simulink model "TorqueDistribution"  (R2024b)
settings: Solver=FixedStepDiscrete  StartTime=0.0  StopTime=1  FixedStep=0.001  RelTol=1e-3  EnableMultiTasking=on
undefined symbols (not defined in the file): MMotorMinAllowed, MTotalMinAllowed, rGearboxRatio, rTyreRadius
libraries: simulink x8
settings Model: DataDictionary=Master_Dictionary.sldd  EnableAccessToBaseWorkspace=off  Creator=torni  LastModifiedBy=oxbro
settings SolverCC: AlgebraicLoopSolver=TrustRegion
settings DataIOCC: ReturnWorkspaceOutputs=off
settings OptimizationCC: DefaultParameterBehavior=Inlined  EnhancedBackFolding=on  PassReuseOutputArgsAs=Individual arguments  ZeroExternalMemoryAtStartup=off  ZeroInternalMemoryAtStartup=off  MaxStackSize=512  OptimizeBlockOrder=speed  DifferentSizesBufferReuse=on  OptimizationCustomize=off  EfficientTunableParamExpr=on
settings DebuggingCC: ParameterTunabilityLossMsg=error  UnconnectedInputMsg=warning  UnconnectedOutputMsg=warning  UnconnectedLineMsg=warning  ArithmeticOperatorsInVariantConditions=warning
settings HardwareCC: ProdBitPerPointer=32  ProdBitPerSizeT=32  ProdBitPerPtrDiffT=32  ProdLargestAtomicInteger=Long  ProdLargestAtomicFloat=Double  ProdWordSize=32  ProdLongLongMode=on  ProdHWDeviceType=ARM Compatible->ARM Cortex-M
settings ModelReferenceCC: EnableRefExpFcnMdlSchedulingChecks=on
settings SFSimCC: MATLABDynamicMemAlloc=off  CustomCodeUndefinedFunction=UseInterfaceOnly
settings RTWCC: Description=Embedded Coder  SystemTargetFile=ert.tlc  HardwareBoard=STM32H7xx Based (Single-core)  TemplateMakefile=ert_default_tmf  CustomHeaderCode="#include \"stm32h7xx_ll_tim.h\""  CustomInitializer=LL_TIM_EnableCounter(TIM2);  Toolchain=GNU Tools for ARM Embedded Processors  GPUComputeCapability=3.5
settings CodeAppCC: ForceParamTrailComments=on  IgnoreCustomStorageClasses=off  OperatorAnnotations=on  SimulinkDataObjDesc=on  SFDataObjDesc=on  InsertBlockDesc=on
settings ERTTargetCC: TargetLangStandard=C99 (ISO)  CodeReplacementLibrary=ARM Cortex-M  ExtModeTransport=3  ExtModeStaticAlloc=on  ExtModeStaticAllocSize=2048  ExtModeMexFile=ext_xcp  ExtModeIntrfLevel=Level2 - Open

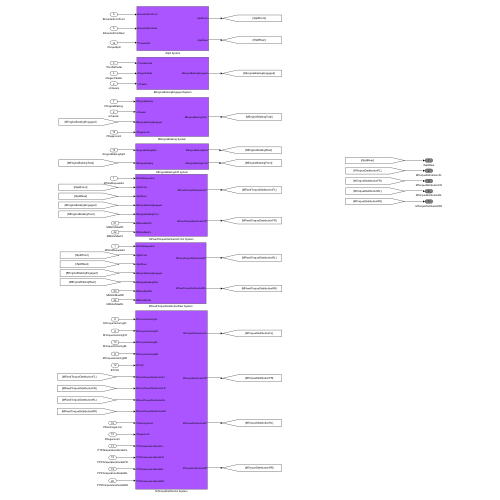
[thumbnail: Simulink's stored preview of the top-level diagram]
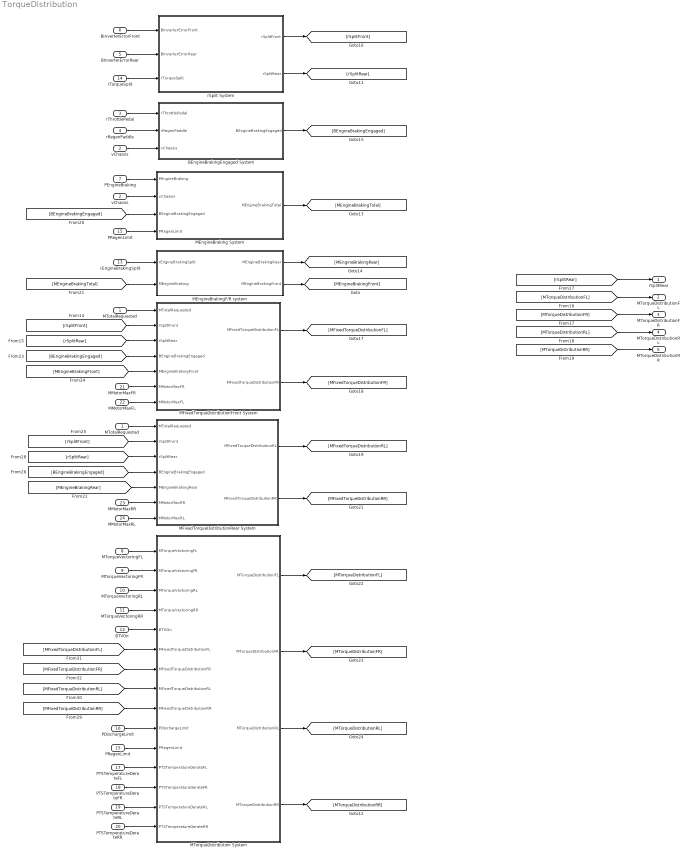
== system TorqueDistribution ==
  MTotalRequested : Inport  OutDataTypeStr=double
  vChassis : Inport  Port=2  OutDataTypeStr=double
  "rThrottlePedal " : Inport  Port=3  OutDataTypeStr=double
  rRegenPaddle : Inport  Port=4  OutDataTypeStr=double
  BInverterErrorRear : Inport  Port=5  OutDataTypeStr=boolean
  BInverterErrorFront : Inport  Port=6  OutDataTypeStr=boolean
  PEngineBraking : Inport  Port=7  OutDataTypeStr=double
  MTorqueVectoringFL : Inport  Port=8  OutDataTypeStr=double
  MTorqueVectoringFR : Inport  Port=9  OutDataTypeStr=double
  MTorqueVectoringRL : Inport  Port=10  OutDataTypeStr=double
  MTorqueVectoringRR : Inport  Port=11  OutDataTypeStr=double
  BTVOn : Inport  Port=12  OutDataTypeStr=boolean
  "rEngineBrakingSplit " : Inport  Port=13
  rTorqueSplit : Inport  Port=14  OutDataTypeStr=double
  PRegenLimit : Inport  Port=15  OutDataTypeStr=double
  PDischargeLimit : Inport  Port=16  OutDataTypeStr=double
  PTSTemperatureDerateFL : Inport  Port=17  OutDataTypeStr=double
  PTSTemperatureDerateFR : Inport  Port=18  OutDataTypeStr=double
  PTSTemperatureDerateRL : Inport  Port=19  OutDataTypeStr=double
  PTSTemperatureDerateRR : Inport  Port=20  OutDataTypeStr=double
  MMotorMaxFR : Inport  Port=21  OutDataTypeStr=double
  MMotorMaxFL : Inport  Port=22  OutDataTypeStr=double
  MMotorMaxRR : Inport  Port=23  OutDataTypeStr=double
  MMotorMaxRL : Inport  Port=24  OutDataTypeStr=double
  BEngineBrakingEngaged System : Subsystem
  MEngineBraking System : Subsystem
  MEngineBrakingF/R system : Subsystem
  MFixedTorqueDistributionFront System : Subsystem
  MFixedTorqueDistributionRear System : Subsystem
  MTorqueDistribution System : Subsystem
  "MTotalRequested " : InportShadow  OutDataTypeStr=double
  "PRegenLimit " : InportShadow  Port=15  OutDataTypeStr=double
  rSplit System : Subsystem
  "vChassis " : InportShadow  Port=2  OutDataTypeStr=double
  rSplitRear : Outport  OutDataTypeStr=double  VectorParamsAs1DForOutWhenUnconnected=off
  MTorqueDistributionFL : Outport  Port=2  OutDataTypeStr=double  VectorParamsAs1DForOutWhenUnconnected=off
  MTorqueDistributionFR : Outport  Port=3  OutDataTypeStr=double  VectorParamsAs1DForOutWhenUnconnected=off
  MTorqueDistributionRL : Outport  Port=4  OutDataTypeStr=double  VectorParamsAs1DForOutWhenUnconnected=off
  MTorqueDistributionRR : Outport  Port=5  OutDataTypeStr=double  VectorParamsAs1DForOutWhenUnconnected=off
  wires:
  [BEngineBrakingEngaged] -> MEngineBraking System/3(BEngineBrakingEngaged)
  vChassis/1 -> BEngineBrakingEngaged System/3(vChassis)
  MEngineBraking System/1("MEngineBrakingTotal ") -> [MEngineBrakingTotal]
  [MEngineBrakingRear] -> MFixedTorqueDistributionRear System/5("MEngineBrakingRear ")
  PEngineBraking/1 -> MEngineBraking System/1(PEngineBraking)
  [MEngineBrakingTotal] -> MEngineBrakingF/R system/2(MEngineBraking)
  MTorqueDistribution System/4(MTorqueDistributionRR) -> [MTorqueDistributionRR]
  [MFixedTorqueDistributionFR] -> MTorqueDistribution System/7(MFixedTorqueDistributionFR)
  MTorqueVectoringFR/1 -> MTorqueDistribution System/2(MTorqueVectoringFR)
  MFixedTorqueDistributionRear System/1(MFixedTorqueDistributionRL) -> [MFixedTorqueDistributionRL]
  [MTorqueDistributionRR] -> MTorqueDistributionRR/1
  "rEngineBrakingSplit "/1 -> MEngineBrakingF/R system/1(rEngineBrakingSplit)
  rTorqueSplit/1 -> rSplit System/3(rTorqueSplit)
  PRegenLimit/1 -> MEngineBraking System/4(PRegenLimit)
  [MTorqueDistributionFL] -> MTorqueDistributionFL/1
  [rSplitRear] -> MFixedTorqueDistributionRear System/3(rSplitRear)
  MEngineBrakingF/R system/1(MEngineBrakingRear) -> [MEngineBrakingRear]
  [rSplitRear] -> MFixedTorqueDistributionFront System/3(rSplitRear)
  BInverterErrorRear/1 -> rSplit System/2(BInverterErrorRear)
  [MTorqueDistributionRL] -> MTorqueDistributionRL/1
  MFixedTorqueDistributionFront System/2(MFixedTorqueDistributionFR) -> [MFixedTorqueDistributionFR]
  MTorqueDistribution System/3(MTorqueDistributionRL) -> [MTorqueDistributionRL]
  [BEngineBrakingEngaged] -> MFixedTorqueDistributionFront System/4(BEngineBrakingEngaged)
  [MFixedTorqueDistributionRR] -> MTorqueDistribution System/9(MFixedTorqueDistributionRR)
  [MTorqueDistributionFR] -> MTorqueDistributionFR/1
  MTorqueDistribution System/2(MTorqueDistributionFR) -> [MTorqueDistributionFR]
  MFixedTorqueDistributionRear System/2(MFixedTorqueDistributionRR) -> [MFixedTorqueDistributionRR]
  [rSplitFront] -> MFixedTorqueDistributionRear System/2(rSplitFront)
  BEngineBrakingEngaged System/1(BEngineBrakingEngaged) -> [BEngineBrakingEngaged]
  "MTotalRequested "/1 -> MFixedTorqueDistributionRear System/1(MTotalRequested)
  rRegenPaddle/1 -> BEngineBrakingEngaged System/2(rRegenPaddle)
  [rSplitFront] -> MFixedTorqueDistributionFront System/2(rSplitFront)
  MTotalRequested/1 -> MFixedTorqueDistributionFront System/1(MTotalRequested)
  "rThrottlePedal "/1 -> BEngineBrakingEngaged System/1("rThrottlePedal ")
  [MFixedTorqueDistributionFL] -> MTorqueDistribution System/6(MFixedTorqueDistributionFL)
  BInverterErrorFront/1 -> rSplit System/1(BInverterErrorFront)
  rSplit System/2(rSplitRear) -> [rSplitRear]
  "vChassis "/1 -> MEngineBraking System/2(vChassis)
  MTorqueVectoringRR/1 -> MTorqueDistribution System/4(MTorqueVectoringRR)
  MTorqueVectoringRL/1 -> MTorqueDistribution System/3(MTorqueVectoringRL)
  MEngineBrakingF/R system/2(MEngineBrakingFront) -> [MEngineBrakingFront]
  [BEngineBrakingEngaged] -> MFixedTorqueDistributionRear System/4(BEngineBrakingEngaged)
  [rSplitRear] -> rSplitRear/1
  [MEngineBrakingFront] -> MFixedTorqueDistributionFront System/5("MEngineBrakingFront ")
  rSplit System/1(rSplitFront) -> [rSplitFront]
  MFixedTorqueDistributionFront System/1(MFixedTorqueDistributionFL) -> [MFixedTorqueDistributionFL]
  MTorqueDistribution System/1(MTorqueDistributionFL) -> [MTorqueDistributionFL]
  BTVOn/1 -> MTorqueDistribution System/5(BTVOn)
  [MFixedTorqueDistributionRL] -> MTorqueDistribution System/8(MFixedTorqueDistributionRL)
  MTorqueVectoringFL/1 -> MTorqueDistribution System/1(MTorqueVectoringFL)
  "PRegenLimit "/1 -> MTorqueDistribution System/11(PRegenLimit)
  PDischargeLimit/1 -> MTorqueDistribution System/10(PDischargeLimit)
  PTSTemperatureDerateFL/1 -> MTorqueDistribution System/12(PTSTemperatureDerateFL)
  PTSTemperatureDerateRR/1 -> MTorqueDistribution System/15(PTSTemperatureDerateRR)
  PTSTemperatureDerateRL/1 -> MTorqueDistribution System/14(PTSTemperatureDerateRL)
  PTSTemperatureDerateFR/1 -> MTorqueDistribution System/13(PTSTemperatureDerateFR)
  MMotorMaxFR/1 -> MFixedTorqueDistributionFront System/6(MMotorMaxFR)
  MMotorMaxFL/1 -> MFixedTorqueDistributionFront System/7(MMotorMaxFL)
  MMotorMaxRR/1 -> MFixedTorqueDistributionRear System/6(MMotorMaxRR)
  MMotorMaxRL/1 -> MFixedTorqueDistributionRear System/7(MMotorMaxRL)

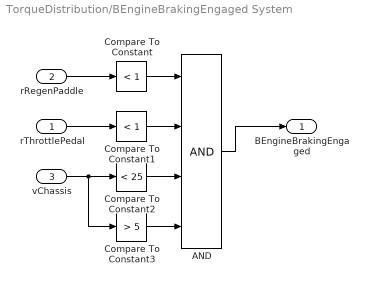
== system TorqueDistribution/BEngineBrakingEngaged System ==
  "rThrottlePedal " : Inport  OutDataTypeStr=double
  rRegenPaddle : Inport  Port=2  OutDataTypeStr=double
  vChassis : Inport  Port=3  OutDataTypeStr=double
  AND : Logic  Inputs=4  AllPortsSameDT=off  OutDataTypeStr=boolean
  Compare To Constant : simulink/Logic and Bit Operations/Compare To Constant  relop=<  const=1  OutDataTypeStr=boolean
  Compare To Constant1 : simulink/Logic and Bit Operations/Compare To Constant  relop=<  const=1  OutDataTypeStr=boolean
  Compare To Constant2 : simulink/Logic and Bit Operations/Compare To Constant  relop=<  const=25  OutDataTypeStr=boolean
  Compare To Constant3 : simulink/Logic and Bit Operations/Compare To Constant  relop=>  const=5  OutDataTypeStr=boolean
  BEngineBrakingEngaged : Outport  OutDataTypeStr=boolean  VectorParamsAs1DForOutWhenUnconnected=off
  wires:
  AND/1 -> BEngineBrakingEngaged/1
  rRegenPaddle/1 -> Compare To Constant/1
  Compare To Constant1/1 -> AND/2
  Compare To Constant/1 -> AND/1
  "rThrottlePedal "/1 -> Compare To Constant1/1
  vChassis/1 -> Compare To Constant3/1, Compare To Constant2/1
  Compare To Constant2/1 -> AND/3
  Compare To Constant3/1 -> AND/4

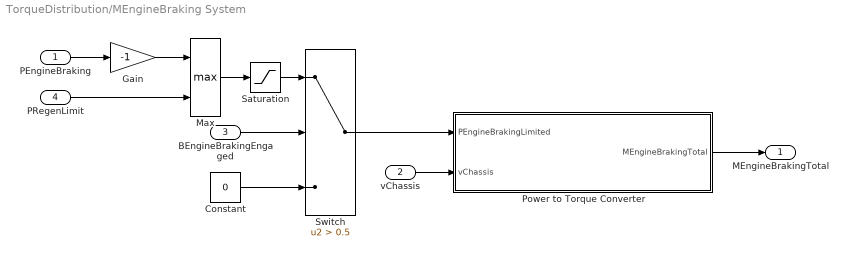
== system TorqueDistribution/MEngineBraking System ==
  PEngineBraking : Inport  OutDataTypeStr=double
  vChassis : Inport  Port=2  OutDataTypeStr=double
  BEngineBrakingEngaged : Inport  Port=3  OutDataTypeStr=boolean
  PRegenLimit : Inport  Port=4  OutDataTypeStr=double
  Constant : Constant  Value=0
  Gain : Gain  Gain=-1
  Max : MinMax  Function=max  Inputs=2
  Power to Torque Converter : Subsystem
  Saturation : Saturate  UpperLimit=0  LowerLimit=-100
  Switch : Switch  Criteria=u2 > Threshold  Threshold=0.5  SaturateOnIntegerOverflow=off  InputSameDT=off
  "MEngineBrakingTotal " : Outport  OutDataTypeStr=double  VectorParamsAs1DForOutWhenUnconnected=off
  wires:
  vChassis/1 -> Power to Torque Converter/2(vChassis)
  PEngineBraking/1 -> Gain/1
  PRegenLimit/1 -> Max/2
  Max/1 -> Saturation/1
  Constant/1 -> Switch/3
  BEngineBrakingEngaged/1 -> Switch/2
  Switch/1 -> Power to Torque Converter/1("PEngineBrakingLimited ")
  Power to Torque Converter/1(MEngineBrakingTotal) -> "MEngineBrakingTotal "/1
  Gain/1 -> Max/1
  Saturation/1 -> Switch/1

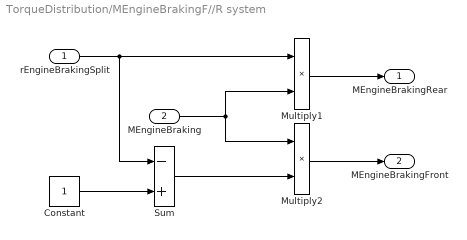
== system TorqueDistribution/MEngineBrakingF//R system ==
  rEngineBrakingSplit : Inport
  MEngineBraking : Inport  Port=2
  Constant : Constant
  Multiply1 : Product
  Multiply2 : Product
  Sum : Sum  Inputs=-+
  MEngineBrakingRear : Outport  VectorParamsAs1DForOutWhenUnconnected=off
  MEngineBrakingFront : Outport  Port=2  VectorParamsAs1DForOutWhenUnconnected=off
  wires:
  Multiply1/1 -> MEngineBrakingRear/1
  MEngineBraking/1 -> Multiply2/1, Multiply1/2
  Multiply2/1 -> MEngineBrakingFront/1
  rEngineBrakingSplit/1 -> Sum/1, Multiply1/1
  Constant/1 -> Sum/2
  Sum/1 -> Multiply2/2

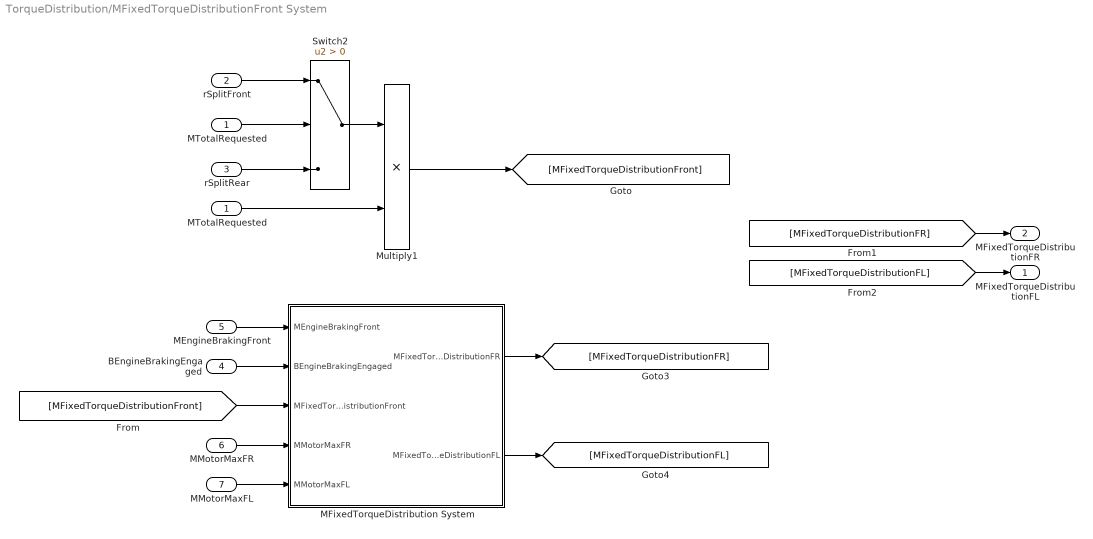
== system TorqueDistribution/MFixedTorqueDistributionFront System ==
  MTotalRequested : Inport  OutDataTypeStr=double
  rSplitFront : Inport  Port=2  OutDataTypeStr=double
  rSplitRear : Inport  Port=3  OutDataTypeStr=double
  BEngineBrakingEngaged : Inport  Port=4  OutDataTypeStr=boolean
  "MEngineBrakingFront " : Inport  Port=5
  MMotorMaxFR : Inport  Port=6  OutDataTypeStr=double
  MMotorMaxFL : Inport  Port=7  OutDataTypeStr=double
  MFixedTorqueDistribution System : Subsystem
  "MTotalRequested " : InportShadow  OutDataTypeStr=double
  Multiply1 : Product
  Switch2 : Switch  Criteria=u2 > Threshold  SaturateOnIntegerOverflow=off  InputSameDT=off
  MFixedTorqueDistributionFL : Outport  VectorParamsAs1DForOutWhenUnconnected=off
  MFixedTorqueDistributionFR : Outport  Port=2  VectorParamsAs1DForOutWhenUnconnected=off
  wires:
  Switch2/1 -> Multiply1/1
  MTotalRequested/1 -> Switch2/2
  rSplitFront/1 -> Switch2/1
  rSplitRear/1 -> Switch2/3
  "MTotalRequested "/1 -> Multiply1/2
  Multiply1/1 -> [MFixedTorqueDistributionFront]
  MFixedTorqueDistribution System/2(MFixedTorqueDistributionFL) -> [MFixedTorqueDistributionFL]
  MFixedTorqueDistribution System/1(MFixedTorqueDistributionFR) -> [MFixedTorqueDistributionFR]
  BEngineBrakingEngaged/1 -> MFixedTorqueDistribution System/2(BEngineBrakingEngaged)
  [MFixedTorqueDistributionFront] -> MFixedTorqueDistribution System/3(MFixedTorqueDistributionFront)
  "MEngineBrakingFront "/1 -> MFixedTorqueDistribution System/1(MEngineBrakingFront)
  [MFixedTorqueDistributionFR] -> MFixedTorqueDistributionFR/1
  [MFixedTorqueDistributionFL] -> MFixedTorqueDistributionFL/1
  MMotorMaxFR/1 -> MFixedTorqueDistribution System/4(MMotorMaxFR)
  MMotorMaxFL/1 -> MFixedTorqueDistribution System/5(MMotorMaxFL)

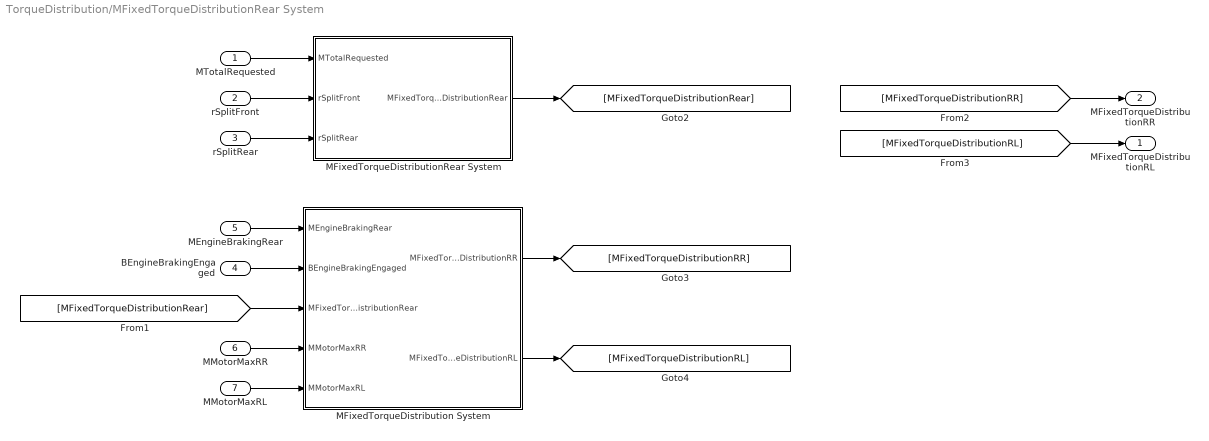
== system TorqueDistribution/MFixedTorqueDistributionRear System ==
  MTotalRequested : Inport  OutDataTypeStr=double
  rSplitFront : Inport  Port=2  OutDataTypeStr=double
  rSplitRear : Inport  Port=3  OutDataTypeStr=double
  BEngineBrakingEngaged : Inport  Port=4  OutDataTypeStr=boolean
  "MEngineBrakingRear " : Inport  Port=5
  MMotorMaxRR : Inport  Port=6  OutDataTypeStr=double
  MMotorMaxRL : Inport  Port=7  OutDataTypeStr=double
  MFixedTorqueDistribution System : Subsystem
  MFixedTorqueDistributionRear System : Subsystem
  MFixedTorqueDistributionRL : Outport  OutDataTypeStr=double  VectorParamsAs1DForOutWhenUnconnected=off
  MFixedTorqueDistributionRR : Outport  Port=2  OutDataTypeStr=double  VectorParamsAs1DForOutWhenUnconnected=off
  wires:
  MTotalRequested/1 -> MFixedTorqueDistributionRear System/1(MTotalRequested)
  rSplitFront/1 -> MFixedTorqueDistributionRear System/2(rSplitFront)
  rSplitRear/1 -> MFixedTorqueDistributionRear System/3(rSplitRear)
  MFixedTorqueDistributionRear System/1(MFixedTorqueDistributionRear) -> [MFixedTorqueDistributionRear]
  BEngineBrakingEngaged/1 -> MFixedTorqueDistribution System/2(BEngineBrakingEngaged)
  "MEngineBrakingRear "/1 -> MFixedTorqueDistribution System/1(MEngineBrakingRear)
  [MFixedTorqueDistributionRear] -> MFixedTorqueDistribution System/3(MFixedTorqueDistributionRear)
  MFixedTorqueDistribution System/1(MFixedTorqueDistributionRR) -> [MFixedTorqueDistributionRR]
  MFixedTorqueDistribution System/2(MFixedTorqueDistributionRL) -> [MFixedTorqueDistributionRL]
  [MFixedTorqueDistributionRR] -> MFixedTorqueDistributionRR/1
  [MFixedTorqueDistributionRL] -> MFixedTorqueDistributionRL/1
  MMotorMaxRR/1 -> MFixedTorqueDistribution System/4(MMotorMaxRR)
  MMotorMaxRL/1 -> MFixedTorqueDistribution System/5(MMotorMaxRL)

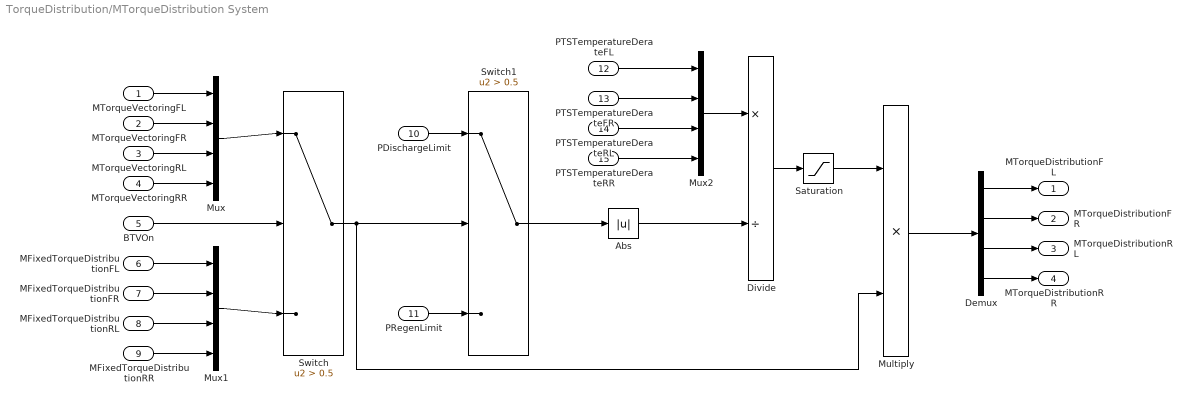
== system TorqueDistribution/MTorqueDistribution System ==
  MTorqueVectoringFL : Inport  OutDataTypeStr=double
  MTorqueVectoringFR : Inport  Port=2  OutDataTypeStr=double
  MTorqueVectoringRL : Inport  Port=3  OutDataTypeStr=double
  MTorqueVectoringRR : Inport  Port=4  OutDataTypeStr=double
  BTVOn : Inport  Port=5  OutDataTypeStr=boolean
  MFixedTorqueDistributionFL : Inport  Port=6  OutDataTypeStr=double
  MFixedTorqueDistributionFR : Inport  Port=7  OutDataTypeStr=double
  MFixedTorqueDistributionRL : Inport  Port=8  OutDataTypeStr=double
  MFixedTorqueDistributionRR : Inport  Port=9  OutDataTypeStr=double
  PDischargeLimit : Inport  Port=10  OutDataTypeStr=double
  PRegenLimit : Inport  Port=11  OutDataTypeStr=double
  PTSTemperatureDerateFL : Inport  Port=12  OutDataTypeStr=double
  PTSTemperatureDerateFR : Inport  Port=13  OutDataTypeStr=double
  PTSTemperatureDerateRL : Inport  Port=14  OutDataTypeStr=double
  PTSTemperatureDerateRR : Inport  Port=15  OutDataTypeStr=double
  Abs : Abs  SaturateOnIntegerOverflow=off
  Demux : Demux
  Divide : Product  Inputs=*/  RndMeth=Zero  SaturateOnIntegerOverflow=on
  Multiply : Product
  Mux : Mux
  Mux1 : Mux
  Mux2 : Mux
  Saturation : Saturate  UpperLimit=1  LowerLimit=0
  Switch : Switch  Criteria=u2 > Threshold  Threshold=0.5  OutDataTypeStr=double  SaturateOnIntegerOverflow=off  InputSameDT=off
  Switch1 : Switch  Criteria=u2 > Threshold  Threshold=0.5  OutDataTypeStr=double  SaturateOnIntegerOverflow=off  InputSameDT=off
  MTorqueDistributionFL : Outport  OutDataTypeStr=double  VectorParamsAs1DForOutWhenUnconnected=off
  MTorqueDistributionFR : Outport  Port=2  OutDataTypeStr=double  VectorParamsAs1DForOutWhenUnconnected=off
  MTorqueDistributionRL : Outport  Port=3  OutDataTypeStr=double  VectorParamsAs1DForOutWhenUnconnected=off
  MTorqueDistributionRR : Outport  Port=4  OutDataTypeStr=double  VectorParamsAs1DForOutWhenUnconnected=off
  wires:
  Demux/2 -> MTorqueDistributionFR/1
  Demux/3 -> MTorqueDistributionRL/1
  MTorqueVectoringRR/1 -> Mux/4
  MTorqueVectoringFR/1 -> Mux/2
  MTorqueVectoringFL/1 -> Mux/1
  MTorqueVectoringRL/1 -> Mux/3
  Demux/4 -> MTorqueDistributionRR/1
  Demux/1 -> MTorqueDistributionFL/1
  Mux/1 -> Switch/1
  Mux1/1 -> Switch/3
  MFixedTorqueDistributionFL/1 -> Mux1/1
  MFixedTorqueDistributionFR/1 -> Mux1/2
  MFixedTorqueDistributionRL/1 -> Mux1/3
  MFixedTorqueDistributionRR/1 -> Mux1/4
  Switch/1 -> Multiply/2, Switch1/2
  PDischargeLimit/1 -> Switch1/1
  PRegenLimit/1 -> Switch1/3
  Switch1/1 -> Abs/1
  PTSTemperatureDerateFL/1 -> Mux2/1
  PTSTemperatureDerateFR/1 -> Mux2/2
  PTSTemperatureDerateRL/1 -> Mux2/3
  PTSTemperatureDerateRR/1 -> Mux2/4
  Mux2/1 -> Divide/1
  Abs/1 -> Divide/2
  Divide/1 -> Saturation/1
  Saturation/1 -> Multiply/1
  Multiply/1 -> Demux/1
  BTVOn/1 -> Switch/2

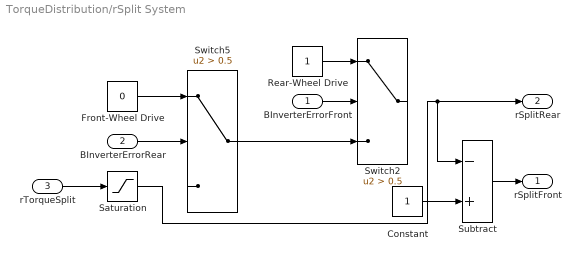
== system TorqueDistribution/rSplit System ==
  BInverterErrorFront : Inport  OutDataTypeStr=boolean
  BInverterErrorRear : Inport  Port=2  OutDataTypeStr=boolean
  rTorqueSplit : Inport  Port=3  OutDataTypeStr=double
  Constant : Constant
  Front-Wheel Drive : Constant  Value=0
  Rear-Wheel Drive : Constant
  Saturation : Saturate  UpperLimit=1  LowerLimit=0
  Subtract : Sum  Inputs=-+
  Switch2 : Switch  Criteria=u2 > Threshold  Threshold=0.5  SaturateOnIntegerOverflow=off  InputSameDT=off
  Switch5 : Switch  Criteria=u2 > Threshold  Threshold=0.5  SaturateOnIntegerOverflow=off  InputSameDT=off
  rSplitFront : Outport  OutDataTypeStr=double  VectorParamsAs1DForOutWhenUnconnected=off
  rSplitRear : Outport  Port=2  OutDataTypeStr=double  VectorParamsAs1DForOutWhenUnconnected=off
  wires:
  BInverterErrorFront/1 -> Switch2/2
  Rear-Wheel Drive/1 -> Switch2/1
  Saturation/1 -> rSplitRear/1, Subtract/1
  Switch5/1 -> Switch2/3
  Front-Wheel Drive/1 -> Switch5/1
  BInverterErrorRear/1 -> Switch5/2
  Subtract/1 -> rSplitFront/1
  Constant/1 -> Subtract/2
  rTorqueSplit/1 -> Saturation/1

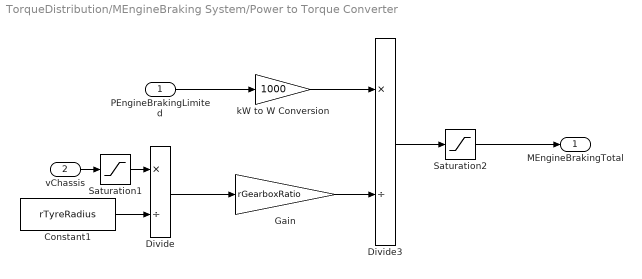
== system TorqueDistribution/MEngineBraking System/Power to Torque Converter ==
  "PEngineBrakingLimited " : Inport
  vChassis : Inport  Port=2  OutDataTypeStr=double
  Constant1 : Constant  Value=rTyreRadius
  Divide : Product  Inputs=*/
  Divide3 : Product  Inputs=*/
  Gain : Gain  Gain=rGearboxRatio
  Saturation1 : Saturate  UpperLimit=40  LowerLimit=0.1
  Saturation2 : Saturate  UpperLimit=0  LowerLimit=MTotalMinAllowed/3
  kW to W Conversion : Gain  Gain=1000
  MEngineBrakingTotal : Outport  OutDataTypeStr=double  VectorParamsAs1DForOutWhenUnconnected=off
  wires:
  "PEngineBrakingLimited "/1 -> kW to W Conversion/1
  Constant1/1 -> Divide/2
  vChassis/1 -> Saturation1/1
  kW to W Conversion/1 -> Divide3/1
  Divide3/1 -> Saturation2/1
  Divide/1 -> Gain/1
  Gain/1 -> Divide3/2
  Saturation1/1 -> Divide/1
  Saturation2/1 -> MEngineBrakingTotal/1

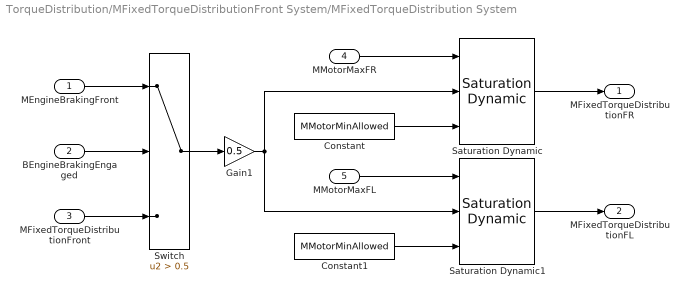
== system TorqueDistribution/MFixedTorqueDistributionFront System/MFixedTorqueDistribution System ==
  MEngineBrakingFront : Inport  OutDataTypeStr=double
  BEngineBrakingEngaged : Inport  Port=2  OutDataTypeStr=boolean
  MFixedTorqueDistributionFront : Inport  Port=3  OutDataTypeStr=double
  MMotorMaxFR : Inport  Port=4  OutDataTypeStr=double
  MMotorMaxFL : Inport  Port=5  OutDataTypeStr=double
  Constant : Constant  Value=MMotorMinAllowed
  Constant1 : Constant  Value=MMotorMinAllowed
  Gain1 : Gain  Gain=0.5
  Saturation Dynamic : simulink/Discontinuities/Saturation Dynamic  OutMin=[]  OutMax=[]  OutDataTypeStr=Inherit: Same as second input  OutDataType=fixdt(1, 16)  OutScaling=2^-10  DoSatur=off
  Saturation Dynamic1 : simulink/Discontinuities/Saturation Dynamic  OutMin=[]  OutMax=[]  OutDataTypeStr=Inherit: Same as second input  OutDataType=fixdt(1, 16)  OutScaling=2^-10  DoSatur=off
  Switch : Switch  Criteria=u2 > Threshold  Threshold=0.5  SaturateOnIntegerOverflow=off  InputSameDT=off
  MFixedTorqueDistributionFR : Outport  OutDataTypeStr=double  VectorParamsAs1DForOutWhenUnconnected=off
  MFixedTorqueDistributionFL : Outport  Port=2  OutDataTypeStr=double  VectorParamsAs1DForOutWhenUnconnected=off
  wires:
  BEngineBrakingEngaged/1 -> Switch/2
  Switch/1 -> Gain1/1
  MFixedTorqueDistributionFront/1 -> Switch/3
  MEngineBrakingFront/1 -> Switch/1
  Gain1/1 -> Saturation Dynamic1/2, Saturation Dynamic/2
  Saturation Dynamic1/1 -> MFixedTorqueDistributionFL/1
  Saturation Dynamic/1 -> MFixedTorqueDistributionFR/1
  Constant/1 -> Saturation Dynamic/3
  MMotorMaxFR/1 -> Saturation Dynamic/1
  Constant1/1 -> Saturation Dynamic1/3
  MMotorMaxFL/1 -> Saturation Dynamic1/1

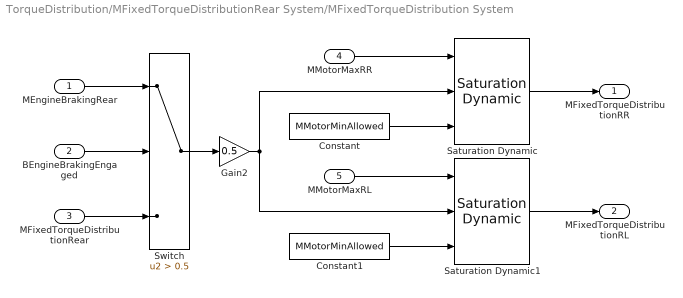
== system TorqueDistribution/MFixedTorqueDistributionRear System/MFixedTorqueDistribution System ==
  MEngineBrakingRear : Inport  OutDataTypeStr=double
  BEngineBrakingEngaged : Inport  Port=2  OutDataTypeStr=boolean
  MFixedTorqueDistributionRear : Inport  Port=3  OutDataTypeStr=double
  MMotorMaxRR : Inport  Port=4  OutDataTypeStr=double
  MMotorMaxRL : Inport  Port=5  OutDataTypeStr=double
  Constant : Constant  Value=MMotorMinAllowed
  Constant1 : Constant  Value=MMotorMinAllowed
  Gain2 : Gain  Gain=0.5
  Saturation Dynamic : simulink/Discontinuities/Saturation Dynamic  OutMin=[]  OutMax=[]  OutDataTypeStr=Inherit: Same as second input  OutDataType=fixdt(1, 16)  OutScaling=2^-10  DoSatur=off
  Saturation Dynamic1 : simulink/Discontinuities/Saturation Dynamic  OutMin=[]  OutMax=[]  OutDataTypeStr=Inherit: Same as second input  OutDataType=fixdt(1, 16)  OutScaling=2^-10  DoSatur=off
  Switch : Switch  Criteria=u2 > Threshold  Threshold=0.5  SaturateOnIntegerOverflow=off  InputSameDT=off
  MFixedTorqueDistributionRR : Outport  OutDataTypeStr=double  VectorParamsAs1DForOutWhenUnconnected=off
  MFixedTorqueDistributionRL : Outport  Port=2  OutDataTypeStr=double  VectorParamsAs1DForOutWhenUnconnected=off
  wires:
  BEngineBrakingEngaged/1 -> Switch/2
  MFixedTorqueDistributionRear/1 -> Switch/3
  MEngineBrakingRear/1 -> Switch/1
  Saturation Dynamic1/1 -> MFixedTorqueDistributionRL/1
  Constant1/1 -> Saturation Dynamic1/3
  MMotorMaxRL/1 -> Saturation Dynamic1/1
  Saturation Dynamic/1 -> MFixedTorqueDistributionRR/1
  Switch/1 -> Gain2/1
  Gain2/1 -> Saturation Dynamic1/2, Saturation Dynamic/2
  Constant/1 -> Saturation Dynamic/3
  MMotorMaxRR/1 -> Saturation Dynamic/1

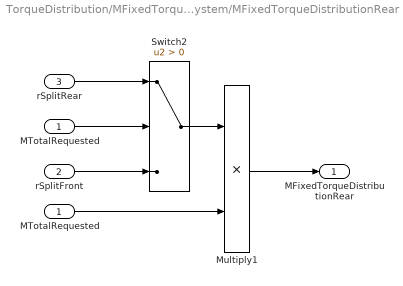
== system TorqueDistribution/MFixedTorqueDistributionRear System/MFixedTorqueDistributionRear System ==
  MTotalRequested : Inport  OutDataTypeStr=double
  rSplitFront : Inport  Port=2  OutDataTypeStr=double
  rSplitRear : Inport  Port=3  OutDataTypeStr=double
  "MTotalRequested " : InportShadow  OutDataTypeStr=double
  Multiply1 : Product
  Switch2 : Switch  Criteria=u2 > Threshold  SaturateOnIntegerOverflow=off  InputSameDT=off
  MFixedTorqueDistributionRear : Outport  OutDataTypeStr=double  VectorParamsAs1DForOutWhenUnconnected=off
  wires:
  rSplitFront/1 -> Switch2/3
  MTotalRequested/1 -> Switch2/2
  "MTotalRequested "/1 -> Multiply1/2
  Switch2/1 -> Multiply1/1
  rSplitRear/1 -> Switch2/1
  Multiply1/1 -> MFixedTorqueDistributionRear/1
